simulink subsystem "CombinedSlipTiresLongitudinal"  (R2024a)
settings: Solver=VariableStepAuto  StartTime=0.0  StopTime=10.0  RelTol=1e-3
undefined symbols (not defined in the file): PlntWhlMaxCmbr, PlntWhlMaxSlipAngle, PlntWhlMaxSlipRatio
libraries: vehdynlibtirecommon x16, vehdynlibtire x4, autolibutils x3
(part 2 of 2)

== system CombinedSlipTiresLongitudinal/Front Friction ==
  u : Inport
  Gain : Gain  Gain=.5
  Selector1 : Selector  InputPortWidth=4  IndexOptions=Index vector (dialog)  Indices=[1 2]  OutputSizes=1
  Sum of Elements : Sum  Inputs=+
  y : Outport
  wires:
  Sum of Elements/1 -> Gain/1
  Gain/1 -> y/1
  Selector1/1 -> Sum of Elements/1
  u/1 -> Selector1/1

== system CombinedSlipTiresLongitudinal/Front Friction1 ==
  u : Inport
  Gain : Gain  Gain=.5
  Selector1 : Selector  InputPortWidth=4  IndexOptions=Index vector (dialog)  Indices=[1 2]  OutputSizes=1
  Sum of Elements : Sum  Inputs=+
  y : Outport
  wires:
  Sum of Elements/1 -> Gain/1
  Gain/1 -> y/1
  Selector1/1 -> Sum of Elements/1
  u/1 -> Selector1/1

== system CombinedSlipTiresLongitudinal/Front Ground ==
  u : Inport
  Gain : Gain  Gain=.5
  Selector1 : Selector  InputPortWidth=4  IndexOptions=Index vector (dialog)  Indices=[1 2]  OutputSizes=1
  Sum of Elements : Sum  Inputs=+
  y : Outport
  wires:
  u/1 -> Selector1/1
  Selector1/1 -> Sum of Elements/1
  Gain/1 -> y/1
  Sum of Elements/1 -> Gain/1

== system CombinedSlipTiresLongitudinal/Front Ground1 ==
  u : Inport
  Gain : Gain  Gain=.5
  Selector1 : Selector  InputPortWidth=4  IndexOptions=Index vector (dialog)  Indices=[1 2]  OutputSizes=1
  Sum of Elements : Sum  Inputs=+
  y : Outport
  wires:
  u/1 -> Selector1/1
  Selector1/1 -> Sum of Elements/1
  Gain/1 -> y/1
  Sum of Elements/1 -> Gain/1

== system CombinedSlipTiresLongitudinal/Rear Friction ==
  u : Inport
  Gain : Gain  Gain=.5
  Selector1 : Selector  InputPortWidth=4  IndexOptions=Index vector (dialog)  Indices=[3 4]  OutputSizes=1
  Sum of Elements : Sum  Inputs=+
  y : Outport
  wires:
  u/1 -> Selector1/1
  Selector1/1 -> Sum of Elements/1
  Gain/1 -> y/1
  Sum of Elements/1 -> Gain/1

== system CombinedSlipTiresLongitudinal/Rear Friction1 ==
  u : Inport
  Gain : Gain  Gain=.5
  Selector1 : Selector  InputPortWidth=4  IndexOptions=Index vector (dialog)  Indices=[3 4]  OutputSizes=1
  Sum of Elements : Sum  Inputs=+
  y : Outport
  wires:
  u/1 -> Selector1/1
  Selector1/1 -> Sum of Elements/1
  Gain/1 -> y/1
  Sum of Elements/1 -> Gain/1

== system CombinedSlipTiresLongitudinal/Rear Ground ==
  u : Inport
  Gain : Gain  Gain=.5
  Selector1 : Selector  InputPortWidth=4  IndexOptions=Index vector (dialog)  Indices=[3 4]  OutputSizes=1
  Sum of Elements : Sum  Inputs=+
  y : Outport
  wires:
  Sum of Elements/1 -> Gain/1
  Gain/1 -> y/1
  Selector1/1 -> Sum of Elements/1
  u/1 -> Selector1/1

== system CombinedSlipTiresLongitudinal/Rear Ground1 ==
  u : Inport
  Gain : Gain  Gain=.5
  Selector1 : Selector  InputPortWidth=4  IndexOptions=Index vector (dialog)  Indices=[3 4]  OutputSizes=1
  Sum of Elements : Sum  Inputs=+
  y : Outport
  wires:
  Sum of Elements/1 -> Gain/1
  Gain/1 -> y/1
  Selector1/1 -> Sum of Elements/1
  u/1 -> Selector1/1

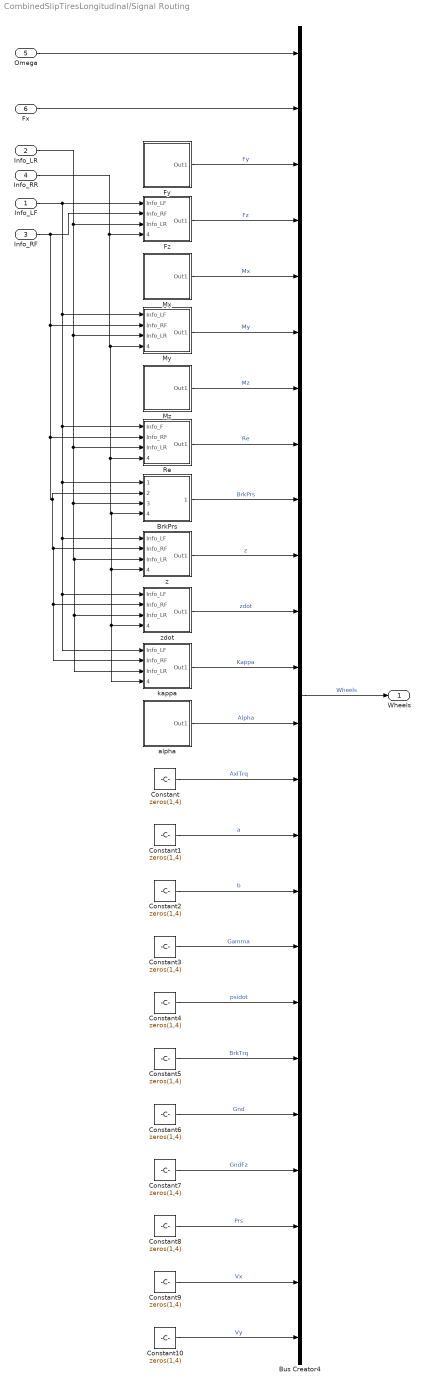
== system CombinedSlipTiresLongitudinal/Signal Routing ==
  Info_LF : Inport
  Info_LR : Inport  Port=2
  Info_RF : Inport  Port=3
  Info_RR : Inport  Port=4
  Omega : Inport  Port=5
  Fx : Inport  Port=6
  BrkPrs : Subsystem
  Bus Creator4 : BusCreator  Inputs=24
  Constant{,1..10} (11 alike) : Constant  Value=zeros(1,4)  SampleTime=-1
  Fy : Subsystem
  Fz : Subsystem
  Mx : Subsystem
  My : Subsystem
  Mz : Subsystem
  Re : Subsystem
  alpha : Subsystem
  kappa : Subsystem
  z : Subsystem
  zdot : Subsystem
  Wheels : Outport
  wires:
  Info_RR/1 -> Fz/4(Info_RR), My/4(Info_RR), BrkPrs/4(Info_RR), z/4(Info_RR), zdot/4(Info_RR), kappa/4(Info_RR), Re/4(Info_RR)
  Info_RF/1 -> Fz/2(Info_RF), My/2(Info_RF), Re/2(Info_RF), BrkPrs/2(Info_RF), z/2(Info_RF), zdot/2(Info_RF), kappa/2(Info_RF)
  Re/1(Out1) -> Bus Creator4/8  "Re"
  Fz/1(Out1) -> Bus Creator4/4  "Fz"
  Info_LF/1 -> BrkPrs/1(Info_LF), zdot/1(Info_LF), kappa/1(Info_LF), z/1(Info_LF), Re/1(Info_F), My/1(Info_LF), Fz/1(Info_LF)
  Info_LR/1 -> BrkPrs/3(Info_LR), kappa/3(Info_LR), zdot/3(Info_LR), z/3(Info_LR), Re/3(Info_LR), My/3(Info_LR), Fz/3(Info_LR)
  Fx/1 -> Bus Creator4/2
  Mx/1(Out1) -> Bus Creator4/5  "Mx"
  zdot/1(Out1) -> Bus Creator4/11  "zdot"
  kappa/1(Out1) -> Bus Creator4/12  "Kappa"
  Mz/1(Out1) -> Bus Creator4/7  "Mz"
  Omega/1 -> Bus Creator4/1
  z/1(Out1) -> Bus Creator4/10  "z"
  Fy/1(Out1) -> Bus Creator4/3  "Fy"
  My/1(Out1) -> Bus Creator4/6  "My"
  alpha/1(Out1) -> Bus Creator4/13  "Alpha"
  Bus Creator4/1 -> Wheels/1  "Wheels"
  BrkPrs/1(BrkPrs) -> Bus Creator4/9  "BrkPrs"
  Constant/1 -> Bus Creator4/14  "AxlTrq"
  Constant1/1 -> Bus Creator4/15  "a"
  Constant2/1 -> Bus Creator4/16  "b"
  Constant3/1 -> Bus Creator4/17  "Gamma"
  Constant4/1 -> Bus Creator4/18  "psidot"
  Constant5/1 -> Bus Creator4/19  "BrkTrq"
  Constant6/1 -> Bus Creator4/20  "Gnd"
  Constant7/1 -> Bus Creator4/21  "GndFz"
  Constant8/1 -> Bus Creator4/22  "Prs"
  Constant9/1 -> Bus Creator4/23  "Vx"
  Constant10/1 -> Bus Creator4/24  "Vy"

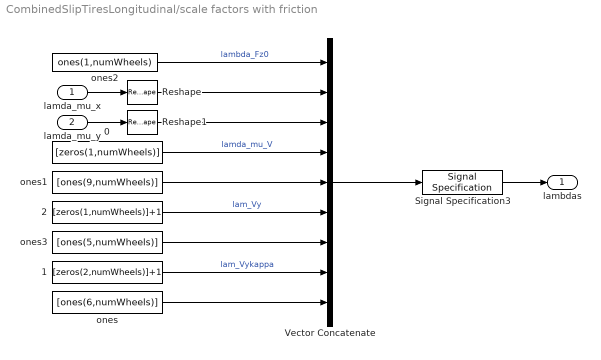
== system CombinedSlipTiresLongitudinal/scale factors with friction ==
  lamda_mu_x : Inport
  lamda_mu_y : Inport  Port=2
  0 : Constant  Value=[zeros(1,numWheels)]  VectorParams1D=off
  1 : Constant  Value=[zeros(2,numWheels)]+1  VectorParams1D=off
  2 : Constant  Value=[zeros(1,numWheels)]+1  VectorParams1D=off
  Reshape : Reshape  OutputDimensionality=Row vector (2-D)  OutputDimensions=[1,numWheels]
  Reshape1 : Reshape  OutputDimensionality=Row vector (2-D)  OutputDimensions=[1,numWheels]
  Signal Specification3 : SignalSpecification  Unit=1
  Vector Concatenate : Concatenate  NumInputs=9  Mode=Multidimensional array
  ones : Constant  Value=[ones(6,numWheels)]  VectorParams1D=off
  ones1 : Constant  Value=[ones(9,numWheels)]  VectorParams1D=off
  ones2 : Constant  Value=ones(1,numWheels)  VectorParams1D=off
  ones3 : Constant  Value=[ones(5,numWheels)]  VectorParams1D=off
  lambdas : Outport  Unit=1  VectorParamsAs1DForOutWhenUnconnected=off
  wires:
  ones3/1 -> Vector Concatenate/7
  2/1 -> Vector Concatenate/6  "lam_Vy"
  ones1/1 -> Vector Concatenate/5
  1/1 -> Vector Concatenate/8  "lam_Vykappa"
  Signal Specification3/1 -> lambdas/1
  Reshape/1 -> Vector Concatenate/2
  Reshape1/1 -> Vector Concatenate/3
  0/1 -> Vector Concatenate/4  "lamda_mu_V"
  ones/1 -> Vector Concatenate/9
  Vector Concatenate/1 -> Signal Specification3/1
  ones2/1 -> Vector Concatenate/1  "lambda_Fz0"
  lamda_mu_x/1 -> Reshape/1
  lamda_mu_y/1 -> Reshape1/1

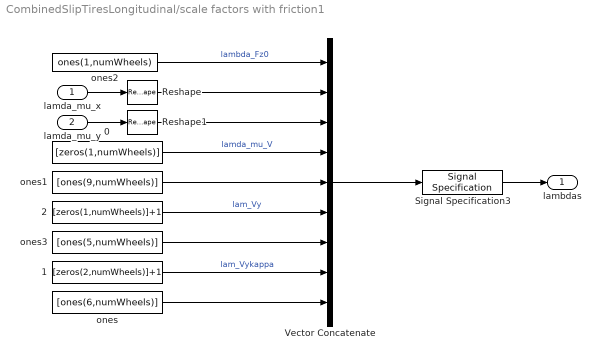
== system CombinedSlipTiresLongitudinal/scale factors with friction1 ==
  lamda_mu_x : Inport
  lamda_mu_y : Inport  Port=2
  0 : Constant  Value=[zeros(1,numWheels)]  VectorParams1D=off
  1 : Constant  Value=[zeros(2,numWheels)]+1  VectorParams1D=off
  2 : Constant  Value=[zeros(1,numWheels)]+1  VectorParams1D=off
  Reshape : Reshape  OutputDimensionality=Row vector (2-D)  OutputDimensions=[1,numWheels]
  Reshape1 : Reshape  OutputDimensionality=Row vector (2-D)  OutputDimensions=[1,numWheels]
  Signal Specification3 : SignalSpecification  Unit=1
  Vector Concatenate : Concatenate  NumInputs=9  Mode=Multidimensional array
  ones : Constant  Value=[ones(6,numWheels)]  VectorParams1D=off
  ones1 : Constant  Value=[ones(9,numWheels)]  VectorParams1D=off
  ones2 : Constant  Value=ones(1,numWheels)  VectorParams1D=off
  ones3 : Constant  Value=[ones(5,numWheels)]  VectorParams1D=off
  lambdas : Outport  Unit=1  VectorParamsAs1DForOutWhenUnconnected=off
  wires:
  lamda_mu_y/1 -> Reshape1/1
  lamda_mu_x/1 -> Reshape/1
  ones2/1 -> Vector Concatenate/1  "lambda_Fz0"
  Vector Concatenate/1 -> Signal Specification3/1
  ones/1 -> Vector Concatenate/9
  0/1 -> Vector Concatenate/4  "lamda_mu_V"
  Reshape1/1 -> Vector Concatenate/3
  Reshape/1 -> Vector Concatenate/2
  Signal Specification3/1 -> lambdas/1
  1/1 -> Vector Concatenate/8  "lam_Vykappa"
  ones1/1 -> Vector Concatenate/5
  2/1 -> Vector Concatenate/6  "lam_Vy"
  ones3/1 -> Vector Concatenate/7

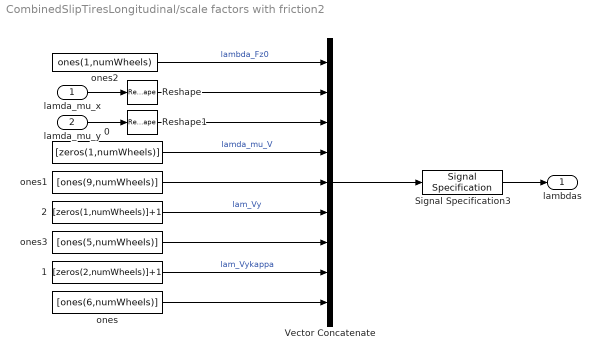
== system CombinedSlipTiresLongitudinal/scale factors with friction2 ==
  lamda_mu_x : Inport
  lamda_mu_y : Inport  Port=2
  0 : Constant  Value=[zeros(1,numWheels)]  VectorParams1D=off
  1 : Constant  Value=[zeros(2,numWheels)]+1  VectorParams1D=off
  2 : Constant  Value=[zeros(1,numWheels)]+1  VectorParams1D=off
  Reshape : Reshape  OutputDimensionality=Row vector (2-D)  OutputDimensions=[1,numWheels]
  Reshape1 : Reshape  OutputDimensionality=Row vector (2-D)  OutputDimensions=[1,numWheels]
  Signal Specification3 : SignalSpecification  Unit=1
  Vector Concatenate : Concatenate  NumInputs=9  Mode=Multidimensional array
  ones : Constant  Value=[ones(6,numWheels)]  VectorParams1D=off
  ones1 : Constant  Value=[ones(9,numWheels)]  VectorParams1D=off
  ones2 : Constant  Value=ones(1,numWheels)  VectorParams1D=off
  ones3 : Constant  Value=[ones(5,numWheels)]  VectorParams1D=off
  lambdas : Outport  Unit=1  VectorParamsAs1DForOutWhenUnconnected=off
  wires:
  ones3/1 -> Vector Concatenate/7
  2/1 -> Vector Concatenate/6  "lam_Vy"
  ones1/1 -> Vector Concatenate/5
  1/1 -> Vector Concatenate/8  "lam_Vykappa"
  Signal Specification3/1 -> lambdas/1
  Reshape/1 -> Vector Concatenate/2
  Reshape1/1 -> Vector Concatenate/3
  0/1 -> Vector Concatenate/4  "lamda_mu_V"
  ones/1 -> Vector Concatenate/9
  Vector Concatenate/1 -> Signal Specification3/1
  ones2/1 -> Vector Concatenate/1  "lambda_Fz0"
  lamda_mu_x/1 -> Reshape/1
  lamda_mu_y/1 -> Reshape1/1

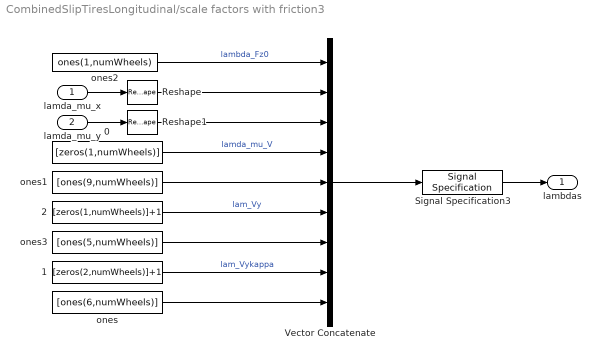
== system CombinedSlipTiresLongitudinal/scale factors with friction3 ==
  lamda_mu_x : Inport
  lamda_mu_y : Inport  Port=2
  0 : Constant  Value=[zeros(1,numWheels)]  VectorParams1D=off
  1 : Constant  Value=[zeros(2,numWheels)]+1  VectorParams1D=off
  2 : Constant  Value=[zeros(1,numWheels)]+1  VectorParams1D=off
  Reshape : Reshape  OutputDimensionality=Row vector (2-D)  OutputDimensions=[1,numWheels]
  Reshape1 : Reshape  OutputDimensionality=Row vector (2-D)  OutputDimensions=[1,numWheels]
  Signal Specification3 : SignalSpecification  Unit=1
  Vector Concatenate : Concatenate  NumInputs=9  Mode=Multidimensional array
  ones : Constant  Value=[ones(6,numWheels)]  VectorParams1D=off
  ones1 : Constant  Value=[ones(9,numWheels)]  VectorParams1D=off
  ones2 : Constant  Value=ones(1,numWheels)  VectorParams1D=off
  ones3 : Constant  Value=[ones(5,numWheels)]  VectorParams1D=off
  lambdas : Outport  Unit=1  VectorParamsAs1DForOutWhenUnconnected=off
  wires:
  lamda_mu_y/1 -> Reshape1/1
  lamda_mu_x/1 -> Reshape/1
  ones2/1 -> Vector Concatenate/1  "lambda_Fz0"
  Vector Concatenate/1 -> Signal Specification3/1
  ones/1 -> Vector Concatenate/9
  0/1 -> Vector Concatenate/4  "lamda_mu_V"
  Reshape1/1 -> Vector Concatenate/3
  Reshape/1 -> Vector Concatenate/2
  Signal Specification3/1 -> lambdas/1
  1/1 -> Vector Concatenate/8  "lam_Vykappa"
  ones1/1 -> Vector Concatenate/5
  2/1 -> Vector Concatenate/6  "lam_Vy"
  ones3/1 -> Vector Concatenate/7

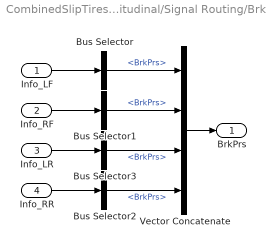
== system CombinedSlipTiresLongitudinal/Signal Routing/BrkPrs ==
  Info_LF : Inport
  Info_RF : Inport  Port=2
  Info_LR : Inport  Port=3
  Info_RR : Inport  Port=4
  Bus Selector{,1..3} (4 alike) : BusSelector  OutputSignals=BrkPrs
  Vector Concatenate : Concatenate  NumInputs=4
  BrkPrs : Outport  PortDimensions=4  VectorParamsAs1DForOutWhenUnconnected=off
  wires:
  Bus Selector2/1 -> Vector Concatenate/4  "<BrkPrs>"
  Info_RR/1 -> Bus Selector2/1
  Bus Selector1/1 -> Vector Concatenate/2  "<BrkPrs>"
  Info_RF/1 -> Bus Selector1/1
  Bus Selector/1 -> Vector Concatenate/1  "<BrkPrs>"
  Info_LF/1 -> Bus Selector/1
  Info_LR/1 -> Bus Selector3/1
  Vector Concatenate/1 -> BrkPrs/1
  Bus Selector3/1 -> Vector Concatenate/3  "<BrkPrs>"

== system CombinedSlipTiresLongitudinal/Signal Routing/Fy ==
  Constant{,1..3} (4 alike) : Constant  Value=0  SampleTime=-1
  Vector Concatenate : Concatenate  NumInputs=4
  Out1 : Outport  PortDimensions=4  VectorParamsAs1DForOutWhenUnconnected=off
  wires:
  Constant/1 -> Vector Concatenate/1  "Fy"
  Vector Concatenate/1 -> Out1/1
  Constant1/1 -> Vector Concatenate/2  "Fy"
  Constant2/1 -> Vector Concatenate/3  "Fy"
  Constant3/1 -> Vector Concatenate/4  "Fy"

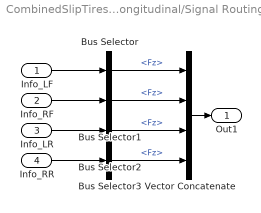
== system CombinedSlipTiresLongitudinal/Signal Routing/Fz ==
  Info_LF : Inport
  Info_RF : Inport  Port=2
  Info_LR : Inport  Port=3
  Info_RR : Inport  Port=4
  Bus Selector{,1..3} (4 alike) : BusSelector  OutputSignals=Fz
  Vector Concatenate : Concatenate  NumInputs=4
  Out1 : Outport  PortDimensions=4  VectorParamsAs1DForOutWhenUnconnected=off
  wires:
  Bus Selector3/1 -> Vector Concatenate/4  "<Fz>"
  Bus Selector2/1 -> Vector Concatenate/3  "<Fz>"
  Bus Selector1/1 -> Vector Concatenate/2  "<Fz>"
  Info_RR/1 -> Bus Selector3/1
  Info_LR/1 -> Bus Selector2/1
  Info_RF/1 -> Bus Selector1/1
  Bus Selector/1 -> Vector Concatenate/1  "<Fz>"
  Info_LF/1 -> Bus Selector/1
  Vector Concatenate/1 -> Out1/1

== system CombinedSlipTiresLongitudinal/Signal Routing/Mx ==
  Constant{,1..3} (4 alike) : Constant  Value=0  SampleTime=-1
  Vector Concatenate : Concatenate  NumInputs=4
  Out1 : Outport  PortDimensions=4  VectorParamsAs1DForOutWhenUnconnected=off
  wires:
  Vector Concatenate/1 -> Out1/1
  Constant1/1 -> Vector Concatenate/2  "Mx"
  Constant/1 -> Vector Concatenate/1  "Mx"
  Constant3/1 -> Vector Concatenate/4  "Mx"
  Constant2/1 -> Vector Concatenate/3  "Mx"

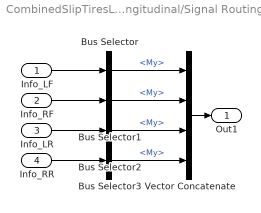
== system CombinedSlipTiresLongitudinal/Signal Routing/My ==
  Info_LF : Inport
  Info_RF : Inport  Port=2
  Info_LR : Inport  Port=3
  Info_RR : Inport  Port=4
  Bus Selector{,1..3} (4 alike) : BusSelector  OutputSignals=My
  Vector Concatenate : Concatenate  NumInputs=4
  Out1 : Outport  PortDimensions=4  VectorParamsAs1DForOutWhenUnconnected=off
  wires:
  Vector Concatenate/1 -> Out1/1
  Info_LF/1 -> Bus Selector/1
  Bus Selector/1 -> Vector Concatenate/1  "<My>"
  Info_RF/1 -> Bus Selector1/1
  Info_LR/1 -> Bus Selector2/1
  Info_RR/1 -> Bus Selector3/1
  Bus Selector1/1 -> Vector Concatenate/2  "<My>"
  Bus Selector2/1 -> Vector Concatenate/3  "<My>"
  Bus Selector3/1 -> Vector Concatenate/4  "<My>"

== system CombinedSlipTiresLongitudinal/Signal Routing/Mz ==
  Constant{,1..3} (4 alike) : Constant  Value=0  SampleTime=-1
  Vector Concatenate : Concatenate  NumInputs=4
  Out1 : Outport  PortDimensions=4  VectorParamsAs1DForOutWhenUnconnected=off
  wires:
  Vector Concatenate/1 -> Out1/1
  Constant1/1 -> Vector Concatenate/2  "Mz"
  Constant/1 -> Vector Concatenate/1  "Mz"
  Constant3/1 -> Vector Concatenate/4  "Mz"
  Constant2/1 -> Vector Concatenate/3  "Mz"

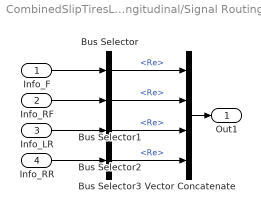
== system CombinedSlipTiresLongitudinal/Signal Routing/Re ==
  Info_F : Inport
  Info_RF : Inport  Port=2
  Info_LR : Inport  Port=3
  Info_RR : Inport  Port=4
  Bus Selector{,1..3} (4 alike) : BusSelector  OutputSignals=Re
  Vector Concatenate : Concatenate  NumInputs=4
  Out1 : Outport  PortDimensions=4  VectorParamsAs1DForOutWhenUnconnected=off
  wires:
  Bus Selector3/1 -> Vector Concatenate/4  "<Re>"
  Bus Selector2/1 -> Vector Concatenate/3  "<Re>"
  Bus Selector1/1 -> Vector Concatenate/2  "<Re>"
  Info_RR/1 -> Bus Selector3/1
  Info_LR/1 -> Bus Selector2/1
  Info_RF/1 -> Bus Selector1/1
  Bus Selector/1 -> Vector Concatenate/1  "<Re>"
  Info_F/1 -> Bus Selector/1
  Vector Concatenate/1 -> Out1/1

== system CombinedSlipTiresLongitudinal/Signal Routing/alpha ==
  Constant{,1..3} (4 alike) : Constant  Value=0  SampleTime=-1
  Vector Concatenate : Concatenate  NumInputs=4
  Out1 : Outport  PortDimensions=4  VectorParamsAs1DForOutWhenUnconnected=off
  wires:
  Vector Concatenate/1 -> Out1/1
  Constant1/1 -> Vector Concatenate/2  "Alpha"
  Constant/1 -> Vector Concatenate/1  "Alpha"
  Constant3/1 -> Vector Concatenate/4  "Alpha"
  Constant2/1 -> Vector Concatenate/3  "Alpha"

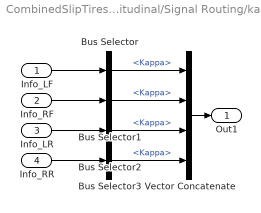
== system CombinedSlipTiresLongitudinal/Signal Routing/kappa ==
  Info_LF : Inport
  Info_RF : Inport  Port=2
  Info_LR : Inport  Port=3
  Info_RR : Inport  Port=4
  Bus Selector{,1..3} (4 alike) : BusSelector  OutputSignals=Kappa
  Vector Concatenate : Concatenate  NumInputs=4
  Out1 : Outport  PortDimensions=4  VectorParamsAs1DForOutWhenUnconnected=off
  wires:
  Vector Concatenate/1 -> Out1/1
  Info_LF/1 -> Bus Selector/1
  Bus Selector/1 -> Vector Concatenate/1  "<Kappa>"
  Info_RF/1 -> Bus Selector1/1
  Info_LR/1 -> Bus Selector2/1
  Info_RR/1 -> Bus Selector3/1
  Bus Selector1/1 -> Vector Concatenate/2  "<Kappa>"
  Bus Selector2/1 -> Vector Concatenate/3  "<Kappa>"
  Bus Selector3/1 -> Vector Concatenate/4  "<Kappa>"

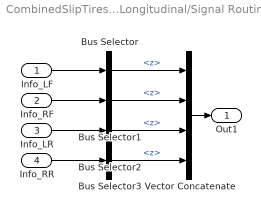
== system CombinedSlipTiresLongitudinal/Signal Routing/z ==
  Info_LF : Inport
  Info_RF : Inport  Port=2
  Info_LR : Inport  Port=3
  Info_RR : Inport  Port=4
  Bus Selector{,1..3} (4 alike) : BusSelector  OutputSignals=z
  Vector Concatenate : Concatenate  NumInputs=4
  Out1 : Outport  PortDimensions=4  VectorParamsAs1DForOutWhenUnconnected=off
  wires:
  Vector Concatenate/1 -> Out1/1
  Info_LF/1 -> Bus Selector/1
  Bus Selector/1 -> Vector Concatenate/1  "<z>"
  Info_RF/1 -> Bus Selector1/1
  Info_LR/1 -> Bus Selector2/1
  Info_RR/1 -> Bus Selector3/1
  Bus Selector1/1 -> Vector Concatenate/2  "<z>"
  Bus Selector2/1 -> Vector Concatenate/3  "<z>"
  Bus Selector3/1 -> Vector Concatenate/4  "<z>"

== system CombinedSlipTiresLongitudinal/Signal Routing/zdot ==
  Info_LF : Inport
  Info_RF : Inport  Port=2
  Info_LR : Inport  Port=3
  Info_RR : Inport  Port=4
  Bus Selector{,1..3} (4 alike) : BusSelector  OutputSignals=zdot
  Vector Concatenate : Concatenate  NumInputs=4
  Out1 : Outport  PortDimensions=4  VectorParamsAs1DForOutWhenUnconnected=off
  wires:
  Bus Selector3/1 -> Vector Concatenate/4  "<zdot>"
  Bus Selector2/1 -> Vector Concatenate/3  "<zdot>"
  Bus Selector1/1 -> Vector Concatenate/2  "<zdot>"
  Info_RR/1 -> Bus Selector3/1
  Info_LR/1 -> Bus Selector2/1
  Info_RF/1 -> Bus Selector1/1
  Bus Selector/1 -> Vector Concatenate/1  "<zdot>"
  Info_LF/1 -> Bus Selector/1
  Vector Concatenate/1 -> Out1/1
